simulink model "udp_com_DCmotor9"  (R2022a)
settings: Solver=VariableStepAuto  StartTime=0.0  StopTime=60  RelTol=1e-3
libraries: spsParallelRLCBranchLib x5, spsGroundLib x5, dspnetwork x5, spsBreakerLib x4, spsCurrentMeasurementLib x3, spsControlledVoltageSourceLib x2, slrealtimeutilitieslib x1, spsSeriesRLCBranchLib x1, spsDCMachineLib x1, spsDCVoltageSourceLib x1, spsIdealSwitchLib x1, spsVoltageMeasurementLib x1
settings Model: Creator=zzh  LastModifiedBy=zzh

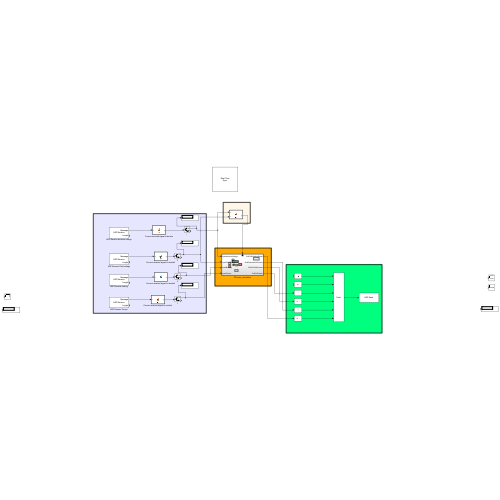
[thumbnail: Simulink's stored preview of the top-level diagram]
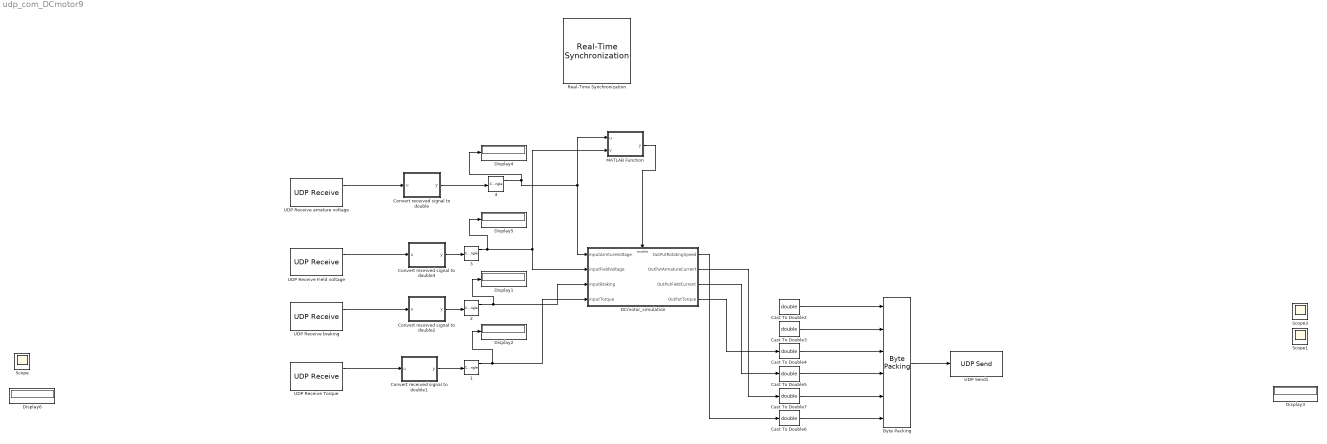
== system udp_com_DCmotor9 ==
  {1..4} (4 alike) : ComplexToMagnitudeAngle
  Byte Packing : slrealtimeutilitieslib/Byte Packing  MaskPackedDataType=double  MaskUnpackedDataTypes={'double','double','double','double','double','double'}  MaskAlignment=1
  Cast To Double{2..7} (6 alike) : DataTypeConversion  OutDataTypeStr=double  SaturateOnIntegerOverflow=off  RndMeth=Floor
  Convert received signal to double : MATLAB Function  TreatAsAtomicUnit=on
  Convert received signal to double1 : MATLAB Function  TreatAsAtomicUnit=on
  Convert received signal to double2 : MATLAB Function  TreatAsAtomicUnit=on
  Convert received signal to double3 : MATLAB Function  TreatAsAtomicUnit=on
  DCmotor_simulation : Subsystem  TreatAsAtomicUnit=on
  Display{1..6} (6 alike) : Display
  MATLAB Function : MATLAB Function  TreatAsAtomicUnit=on
  Real-Time Synchronization : sldrtlib/Real-Time Synchronization  SampleTime=0.01  MaxMissedTicks=100000  ShowMissedTicks=off  YieldWhenWaiting=off
  Scope : Scope
  Scope1 : Scope
  Scope3 : Scope
  UDP Receive Field voltage : dspnetwork/UDP Receive  localURL='0.0.0.0'  localPort=12345  remoteURL='127.0.0.8'  remotePort=-1  recvBufferSize=8192  dims=8192  signalDatatype=uint8  isComplex=off  isVarSize=off  showBlockingTime=off  blockingTime=0  sampletime=0.01  blockPlatform=[]
  UDP Receive Torque : dspnetwork/UDP Receive  localURL='0.0.0.0'  localPort=15555  remoteURL='127.1.1.5'  remotePort=-1  recvBufferSize=8192  dims=8192  signalDatatype=uint8  isComplex=off  isVarSize=off  showBlockingTime=off  blockingTime=0  sampletime=0.01  blockPlatform=[]
  UDP Receive arnature voltage : dspnetwork/UDP Receive  localURL='0.0.0.0'  localPort=12341  remoteURL='127.0.0.5'  remotePort=-1  recvBufferSize=8192  dims=8192  signalDatatype=uint8  isComplex=off  isVarSize=off  showBlockingTime=off  blockingTime=0  sampletime=0.01  blockPlatform=[]
  UDP Receive braking : dspnetwork/UDP Receive  localURL='0.0.0.0'  localPort=12333  remoteURL='127.0.2.5'  remotePort=-1  recvBufferSize=8192  dims=8192  signalDatatype=uint8  isComplex=off  isVarSize=off  showBlockingTime=off  blockingTime=0  sampletime=0.01  blockPlatform=[]
  UDP Send1 : dspnetwork/UDP Send  remoteURL='127.0.5.1'  remotePort=23333  localURL='0.0.0.0'  localPortSource=Automatically determine  localPort=-1  sendBufferSize=8192  sampletime=-1  blockPlatform=[]  separateLengthPort=0
  wires:
  DCmotor_simulation/3(OutPutFieldCurrent) -> Cast To Double5/1
  Cast To Double3/1 -> Byte Packing/2
  Convert received signal to double3/1(y) -> 3/1
  Cast To Double2/1 -> Byte Packing/1
  Byte Packing/1 -> UDP Send1/1
  3/1 -> Display5/1, DCmotor_simulation/2(inputFieldVoltage), MATLAB Function/2(v)
  Cast To Double7/1 -> Byte Packing/5
  Cast To Double4/1 -> Byte Packing/3
  DCmotor_simulation/2(OutPutArmatureCurrent) -> Cast To Double7/1
  Cast To Double6/1 -> Byte Packing/6
  4/1 -> MATLAB Function/1(u), DCmotor_simulation/1(inputArmtureVoltage), Display4/1
  UDP Receive arnature voltage/1 -> Convert received signal to double/1(u)
  Cast To Double5/1 -> Byte Packing/4
  UDP Receive Field voltage/1 -> Convert received signal to double3/1(u)
  DCmotor_simulation/4(OutPutTorque) -> Cast To Double4/1
  Convert received signal to double/1(y) -> 4/1
  DCmotor_simulation/1(OutPutRotatingSpeed) -> Cast To Double6/1
  MATLAB Function/1(y) -> DCmotor_simulation/Enable
  UDP Receive braking/1 -> Convert received signal to double2/1(u)
  Convert received signal to double2/1(y) -> 2/1
  2/1 -> Display1/1, DCmotor_simulation/3(inputBraking)
  1/1 -> Display2/1, DCmotor_simulation/4(inputTorque)
  UDP Receive Torque/1 -> Convert received signal to double1/1(u)
  Convert received signal to double1/1(y) -> 1/1

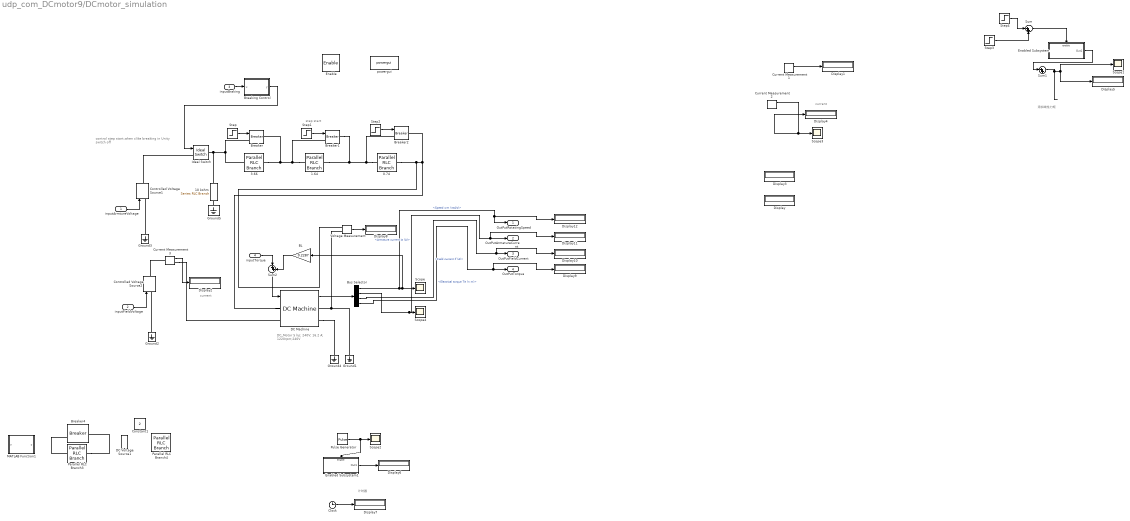
== system udp_com_DCmotor9/DCmotor_simulation ==
  note: DC_Motor
      | 5 hp;  240V;  16.2 A;  1220rpm;240V
  note: 计时器
  note: 添加线性力矩
  note: current
  note: current
  note: control step start,when clike breaking in Unity
      | switch off
  note: step start
  inputArmtureVoltage : Inport
  inputFieldVoltage : Inport  Port=2
  inputBraking : Inport  Port=3
  inputTorque : Inport  Port=4
  Enable : EnablePort  StatesWhenEnabling=reset
  0.74 : spsParallelRLCBranchLib/Parallel RLC Branch  LConnTagsString=a  RConnTagsString=__new0  BranchType=R  Resistance=0.74  Inductance=0  SetiL0=off  InitialCurrent=0  Capacitance=0  Setx0=off  InitialVoltage=0  Measurements=None
  1.64 : spsParallelRLCBranchLib/Parallel RLC Branch  LConnTagsString=a  RConnTagsString=__new0  BranchType=R  Resistance=1.64  Inductance=0  SetiL0=off  InitialCurrent=0  Capacitance=0  Setx0=off  InitialVoltage=0  Measurements=None
  10 kohm : spsSeriesRLCBranchLib/Series RLC Branch  LConnTagsString=__new0  RConnTagsString=__new0  BranchType=R  Resistance=1e4  Inductance=[]  SetiL0=off  InitialCurrent=0  Capacitance=[]  Setx0=off  InitialVoltage=0  Measurements=None
  3.66 : spsParallelRLCBranchLib/Parallel RLC Branch  LConnTagsString=a  RConnTagsString=__new0  BranchType=R  Resistance=3.66  Inductance=0  SetiL0=off  InitialCurrent=0  Capacitance=0  Setx0=off  InitialVoltage=0  Measurements=None
  BL : Gain  Gain=0.2287  SaturateOnIntegerOverflow=on  OutDataTypeStr=Inherit: Same as input  ParamDataTypeStr=Inherit: Same as input
  Breaker : spsBreakerLib/Breaker  InitialState=0  SwitchingTimes="[ 4/60  5/60 ]"  External=on  BreakerResistance=0.01  SnubberResistance=inf  SnubberCapacitance=0  Measurements=None  MoreParameters=off  NoBreakLoop=off
      settings: AttributesFormatString=\n  SourceProductBaseCode=PS
  Breaker1 : spsBreakerLib/Breaker  InitialState=0  SwitchingTimes="[ 4/60  5/60 ]"  External=on  BreakerResistance=0.01  SnubberResistance=inf  SnubberCapacitance=0  Measurements=None  MoreParameters=off  NoBreakLoop=off
      settings: AttributesFormatString=\n  SourceProductBaseCode=PS
  Breaker2 : spsBreakerLib/Breaker  InitialState=0  SwitchingTimes="[ 4/60  5/60 ]"  External=on  BreakerResistance=0.01  SnubberResistance=inf  SnubberCapacitance=0  Measurements=None  MoreParameters=off  NoBreakLoop=off
      settings: AttributesFormatString=\n  SourceProductBaseCode=PS
  Breaker4 : spsBreakerLib/Breaker  InitialState=1  SwitchingTimes="[1/60  5/60]"  External=on  BreakerResistance=0.01  SnubberResistance=1e6  SnubberCapacitance=inf  Measurements=None  MoreParameters=on  NoBreakLoop=off
      settings: SourceProductBaseCode=PS
  Breaking Control : MATLAB Function  TreatAsAtomicUnit=on
  Bus Selector : BusSelector  OutputSignals=Speed wm (rad/s),Armature current ia (A),Field current if (A),Electrical torque Te (n m)
  Clock : Clock
  Constant1 : Constant  Value=2
  Controlled Voltage Source1 : spsControlledVoltageSourceLib/Controlled Voltage Source  Initialize=on  Source_Type=DC  Amplitude=0  Phase=0  Frequency=0  Measurements=Voltage
  Controlled Voltage Source2 : spsControlledVoltageSourceLib/Controlled Voltage Source  Initialize=on  Source_Type=DC  Amplitude=0  Phase=0  Frequency=0  Measurements=Voltage
  Current Measurement1 : spsCurrentMeasurementLib/Current Measurement  PhasorSimulation=off  OutputType=Complex  PSBequivalent=0
  Current Measurement2 : spsCurrentMeasurementLib/Current Measurement  PhasorSimulation=off  OutputType=Complex  PSBequivalent=0
  Current Measurement3 : spsCurrentMeasurementLib/Current Measurement  PhasorSimulation=off  OutputType=Complex  PSBequivalent=0
  DC Machine : spsDCMachineLib/DC Machine  PresetModel=No  MechanicalLoad=Torque TL  FieldType=Wound  ShowDetailedParameters=on  MeasurementBus=off  RLa="[ 0.6  0.012]"  RLf="[ 240  120]"  Laf=1.8  MachineConstant=Torque constant (N.m/A)  Ke=1.8  Kt=1.8  J=1  Bm=0  Tf=0  w0=1  Ifinit=0  TsPowergui=0  TsBlock=-1
  DC Voltage Source1 : spsDCVoltageSourceLib/DC Voltage Source  Amplitude=300  Measurements=Voltage
  Display{,1..12} (13 alike) : Display
  Enabled Subsystem : Subsystem  TreatAsAtomicUnit=on
  Enabled Subsystem1 : Subsystem  TreatAsAtomicUnit=on
  Ground{1..5} (5 alike) : spsGroundLib/Ground  LConnTagsString=a
  Ideal Switch : spsIdealSwitchLib/Ideal Switch  Ron=1e-4  Lon=10e-6  IC=1  Rs=inf  Cs=0  Measurements=off
      settings: AttributesFormatString=\n
  MATLAB Function1 : MATLAB Function  TreatAsAtomicUnit=on
  Parallel RLC Branch3 : spsParallelRLCBranchLib/Parallel RLC Branch  LConnTagsString=a  RConnTagsString=__new0  BranchType=R  Resistance=1  Inductance=0  SetiL0=off  InitialCurrent=0  Capacitance=0  Setx0=off  InitialVoltage=0  Measurements=None
  Parallel RLC Branch4 : spsParallelRLCBranchLib/Parallel RLC Branch  LConnTagsString=a  RConnTagsString=__new0  BranchType=R  Resistance=1000  Inductance=0  SetiL0=off  InitialCurrent=0  Capacitance=0  Setx0=off  InitialVoltage=0  Measurements=None
  Pulse Generator : DiscretePulseGenerator  PulseType=Time based  Period=0.1  PulseWidth=5
  Scope{,1..4} (5 alike) : Scope
  Step : Step  Time=12  SampleTime=0
  Step1 : Step  Time=14  SampleTime=0
  Step2 : Step  Time=16  SampleTime=0
  Step3 : Step  Time=5  SampleTime=0.001
  Step4 : Step  Time=7  After=-1  SampleTime=0.001
  Sum : Sum  Inputs=|++
  Sum1 : Sum  Inputs=|++
  Sum2 : Sum  Inputs=|++
  Voltage Measurement : spsVoltageMeasurementLib/Voltage Measurement  PhasorSimulation=off  OutputType=Complex  PSBequivalent=0
  powergui : spspowerguiLib/powergui  Priority=1  SimulationMode=Discrete  SampleTime=1e-5  frequency=60  Iterations=50  frequencyindice=0  Pbase=100e6  ErrMax=1e-4  UnitsV=kV  UnitsW=MW  buscounter=0  FunctionMessages=off  echomessages=off  EnableUseOfTLC=off  CurrentSourceSwitches=off  DisableSnubberDevices=off  DisableRonSwitches=off  DisableVfSwitches=off  DisplayEquations=off  AutomaticDiscreteSolvers=off  SolverType=Tustin/Backward Euler (TBE)  Interpol=off  ExternalGateDelay=off  methode=off  Ts=100  x0status=blocks  SPID=on  SwTol=0  HookPort=off  NonlinearTolerance=1e-4  nMaxIteration=100  ContinueOnMaxIteration=off  RestoreLinks=warning  ResistiveCurrentMeasurement=off  Frange=[0:2:500]  Ylog=off  Xlog=on  ShowGrid=off  save=off  variable=ZData  structure=0  ZoomFFT=off  StartTime=0.0  cycles=1  DisplayStyle=1  fundamental=60  FreqAxis=off  MaxFrequency=1000  frequencyindicesteady=1  RmsSteady=1  display=off
  OutPutRotatingSpeed : Outport
  OutPutArmatureCurrent : Outport  Port=2
  OutPutFieldCurrent : Outport  Port=3
  OutPutTorque : Outport  Port=4
  wires:
  DC Machine/1 -> Bus Selector/1
  Bus Selector/1 -> BL/1, Scope/1, Display12/1, OutPutRotatingSpeed/1  "<Speed wm (rad/s)>"
  inputArmtureVoltage/1 -> Controlled Voltage Source1/1
  Bus Selector/2 -> Display11/1, OutPutArmatureCurrent/1, Scope4/1  "<Armature current ia (A)>"
  Bus Selector/3 -> Display10/1, OutPutFieldCurrent/1  "<Field current if (A)>"
  Bus Selector/4 -> Display9/1, OutPutTorque/1  "<Electrical torque Te (n m)>"
  inputFieldVoltage/1 -> Controlled Voltage Source2/1
  Current Measurement1/1 -> Display1/1
  Current Measurement2/1 -> Display4/1, Scope3/1
  Current Measurement3/1 -> Display2/1
  Sum1/1 -> Scope1/1, Display5/1
  Sum/1 -> Enabled Subsystem/Enable
  Step4/1 -> Sum/1
  inputTorque/1 -> Sum2/1
  Enabled Subsystem/1(Out1) -> Sum1/1
  Step3/1 -> Sum/2
  Pulse Generator/1 -> Enabled Subsystem1/Enable, Scope2/1
  Enabled Subsystem1/1(Out1) -> Display6/1
  Clock/1 -> Display7/1
  inputBraking/1 -> Breaking Control/1(u)
  Breaking Control/1(y) -> Ideal Switch/1
  Step2/1 -> Breaker2/1
  Step/1 -> Breaker/1
  Step1/1 -> Breaker1/1
  Voltage Measurement/1 -> Display8/1
  BL/1 -> Sum2/2
  Sum2/1 -> DC Machine/1
  connections:
  Current Measurement3/LConn1 -- Controlled Voltage Source2/RConn1
  Ground3/LConn1 -- Controlled Voltage Source1/LConn1
  Ground1/LConn1 -- Voltage Measurement/LConn2 -- DC Machine/RConn1
  Parallel RLC Branch3/LConn1 -- Breaker4/LConn1
  Parallel RLC Branch3/RConn1 -- Breaker4/RConn1
  Ground2/LConn1 -- Controlled Voltage Source2/LConn1
  DC Machine/RConn2 -- Ground4/LConn1
  Current Measurement3/RConn1 -- DC Machine/LConn2
  10 kohm/RConn1 -- Ground5/LConn1
  1.64/LConn1 -- Breaker1/LConn1 -- Breaker/RConn1 -- 3.66/RConn1
  0.74/LConn1 -- Breaker2/LConn1 -- Breaker1/RConn1 -- 1.64/RConn1
  0.74/RConn1 -- Breaker2/RConn1 -- DC Machine/LConn1 -- Voltage Measurement/LConn1
  3.66/LConn1 -- 10 kohm/LConn1 -- Ideal Switch/RConn1 -- Breaker/LConn1
  Controlled Voltage Source1/RConn1 -- Ideal Switch/LConn1

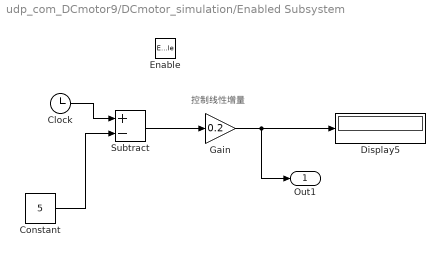
== system udp_com_DCmotor9/DCmotor_simulation/Enabled Subsystem ==
  note: 控制线性增量
  Enable : EnablePort
  Clock : Clock
  Constant : Constant  Value=5
  Display5 : Display
  Gain : Gain  Gain=0.2
  Subtract : Sum  Inputs=+-
  Out1 : Outport
  wires:
  Clock/1 -> Subtract/1
  Constant/1 -> Subtract/2
  Subtract/1 -> Gain/1
  Gain/1 -> Out1/1, Display5/1

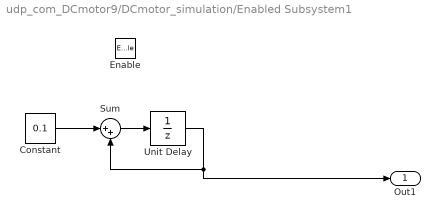
== system udp_com_DCmotor9/DCmotor_simulation/Enabled Subsystem1 ==
  Enable : EnablePort
  Constant : Constant  Value=0.1  SampleTime=0.1
  Sum : Sum  Inputs=|++
  Unit Delay : UnitDelay  SampleTime=-1  HasFrameUpgradeWarning=on
  Out1 : Outport
  wires:
  Constant/1 -> Sum/1
  Sum/1 -> Unit Delay/1
  Unit Delay/1 -> Out1/1, Sum/2

== matlab function udp_com_DCmotor9/Convert received signal to double ==
  data: u input; y output double
function y = fcn(u)

 % 从UDP接收数据
    

    % 将字节数组转换为字符串
    str = char(u);

    % 将字符串转换为数字
    y= str2double(str);
    
end

== matlab function udp_com_DCmotor9/MATLAB Function ==
  data: u input; y output; v input
function y = fcn(u,v)

% 判断输入量是否为空
if v>0.2
    y = 1;
else
    y = 0;
end

== matlab function udp_com_DCmotor9/Convert received signal to double2 ==
  data: u input; y output double
function y = fcn(u)

 % 从UDP接收数据
    

    % 将字节数组转换为字符串
    str = char(u);

    % 将字符串转换为数字
    y= str2double(str);
    
end

== matlab function udp_com_DCmotor9/Convert received signal to double1 ==
  data: u input; y output double
function y = fcn(u)

 % 从UDP接收数据
    

    % 将字节数组转换为字符串
    str = char(u);

    % 将字符串转换为数字
    y= str2double(str);
    
end

== matlab function udp_com_DCmotor9/DCmotor_simulation/MATLAB Function1 ==
  data: u input; y output
function y = fcn(u)

% 判断输入量是否为空
if u>0.01
    y = 0;
else
    y = 1;
end

== matlab function udp_com_DCmotor9/DCmotor_simulation/Breaking Control ==
  data: u input; y output double
function y = fcn(u)

if u==1
    y=0;
else
    y=1;
end
    
end

== matlab function udp_com_DCmotor9/Convert received signal to double3 ==
  data: u input; y output double
function y = fcn(u)

 % 从UDP接收数据
    

    % 将字节数组转换为字符串
    str = char(u);

    % 将字符串转换为数字
    y= str2double(str);
    
end
